simulink model "ccmodel"  (R2023b)
settings: Solver=VariableStepAuto  StartTime=0.0  StopTime=120  RelTol=1e-3
values from neighbouring files (symbols this model uses):
  b = 50    [car.m]    (also in car_PID.m; car_PID_1.m; car_PI_1.m; car_PI_40.m)
  m = 1000    [car.m]    (also in car_PID.m; car_PID_1.m; car_PI_1.m; car_PI_40.m)
settings Model: Creator=user  LastModifiedBy=user

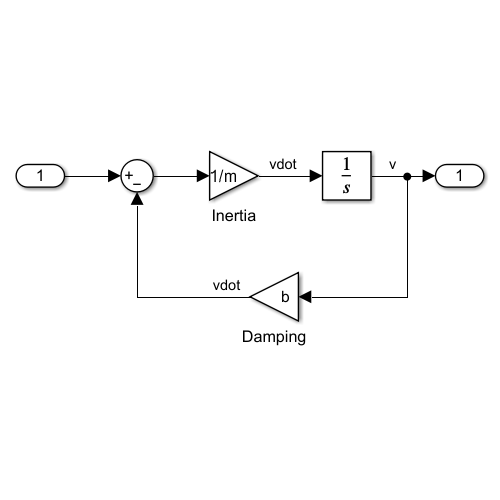
[thumbnail: Simulink's stored preview of the top-level diagram]
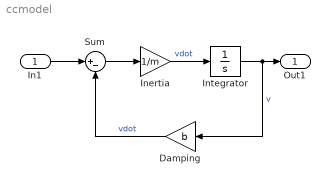
== system ccmodel ==
  In1 : Inport
  Damping : Gain  Gain=b
  Inertia : Gain  Gain=1/m
  Integrator : Integrator
  Sum : Sum  Inputs=|+-
  Out1 : Outport
  wires:
  Inertia/1 -> Integrator/1  "vdot"
  Integrator/1 -> Out1/1, Damping/1  "v"
  Sum/1 -> Inertia/1
  Damping/1 -> Sum/2  "vdot"
  In1/1 -> Sum/1
